simulink library "Min_Stop_Time"  (Simulink 8.2)
settings: Solver=ode45  StartTime=0.0  StopTime=10.0  RelTol=1e-3
libraries: simulink x2
settings Model: Creator=lena.frank  LastModifiedBy=drhf

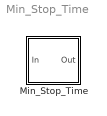
== system Min_Stop_Time ==
  Min_Stop_Time : Subsystem  mask(Minimum Stop Time){tminstop=15}
      mask prompts: tminstop "Minimum stop time in s"
      mask help: Once stopped, the output is held to zero for at least the minimum stop time.
      mask Help: web(fullfile(path_carnot('help'),'Min_Stop_Time.html'),'-helpbrowser')
      mask Display:
      | plot(-20,-30,120,100,[10,20,40,60,80,90,90,80,60,40,20,10,10],[40,20,10,10,20,40,60,80,90,90,80,60,40],[55,46],[95,95],[50,50],[90,95],[50,50,24],[88,50,66],[10,13],[50,50],[90,87],[50,50],[50,50],[10,15])
      | disp('\n\nMin Off')

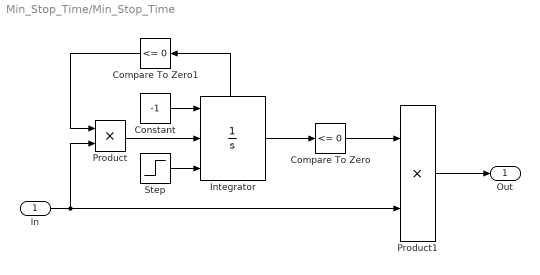
== system Min_Stop_Time/Min_Stop_Time ==
  In : Inport
  Compare To Zero : simulink/Logic and Bit Operations/Compare To Zero  relop=<=  OutDataTypeStr=uint8
  Compare To Zero1 : simulink/Logic and Bit Operations/Compare To Zero  relop=<=  OutDataTypeStr=uint8
  Constant : Constant  Value=-1
  Integrator : Integrator  ExternalReset=falling  InitialConditionSource=external  InitialCondition=tminstop  LimitOutput=on  LowerSaturationLimit=0  ShowStatePort=on
  Product : Product  RndMeth=Zero
  Product1 : Product  RndMeth=Zero
  Step : Step  Time=0.1  After=tminstop  SampleTime=0
  Out : Outport
  wires:
  Constant/1 -> Integrator/1
  Integrator/1 -> Compare To Zero/1
  Compare To Zero/1 -> Product1/1
  In/1 -> Product/2, Product1/2
  Product1/1 -> Out/1
  Product/1 -> Integrator/2
  Integrator/State -> Compare To Zero1/1
  Compare To Zero1/1 -> Product/1
  Step/1 -> Integrator/3
